simulink model "QSMC_TEST"  (R2019a)
settings: Solver=FixedStepAuto  StartTime=0.0  StopTime=10.0  FixedStep=0.02  RelTol=1e-3
settings Model: Creator=anton  LastModifiedBy=anton

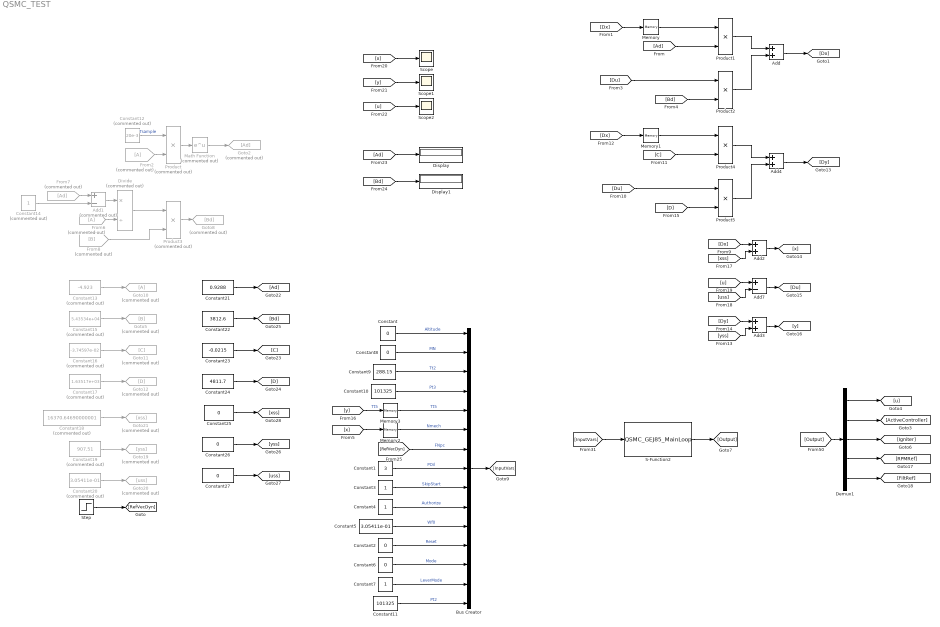
== system QSMC_TEST ==
  Add{,2..4} (4 alike) : Sum
  Add1 : Sum  Commented=on  Inputs=+-
  Add7 : Sum  Inputs=+-
  Bus Creator : BusCreator  Inputs=15
  Constant{,2,6,8,25..27} (7 alike) : Constant  Value=0
  Constant1 : Constant  Value=3
  Constant10 : Constant  Value=101325
  Constant11 : Constant  Value=101325
  Constant12 : Constant  Commented=on  Value=20e-3
  Constant13 : Constant  Commented=on  Value=-4.923
  Constant14 : Constant  Commented=on
  Constant15 : Constant  Commented=on  Value=5.43534e+04
  Constant16 : Constant  Commented=on  Value=-3.74597e-02
  Constant17 : Constant  Commented=on  Value=1.63517e+03
  Constant18 : Constant  Commented=on  Value=16370.64690000001
  Constant19 : Constant  Commented=on  Value=907.51
  Constant20 : Constant  Commented=on  Value=3.05411e-01
  Constant21 : Constant  Value=0.9288
  Constant22 : Constant  Value=3812.6
  Constant23 : Constant  Value=-0.0215
  Constant24 : Constant  Value=4811.7
  Constant3 : Constant
  Constant4 : Constant
  Constant5 : Constant  Value=3.05411e-01
  Constant7 : Constant
  Constant9 : Constant  Value=288.15
  Demux1 : Demux  Outputs=5
  Display : Display
  Display1 : Display
  Divide : Product  Commented=on  Inputs=*/
  From2 : From  Commented=on
  From6 : From  Commented=on
  From7 : From  Commented=on  GotoTag=Ad
  From8 : From  Commented=on  GotoTag=B
  Goto10 : Goto  Commented=on
  Goto11 : Goto  Commented=on  GotoTag=C
  Goto12 : Goto  Commented=on  GotoTag=D
  Goto19 : Goto  Commented=on  GotoTag=yss
  Goto2 : Goto  Commented=on  GotoTag=Ad
  Goto20 : Goto  Commented=on  GotoTag=uss
  Goto21 : Goto  Commented=on  GotoTag=xss
  Goto5 : Goto  Commented=on  GotoTag=B
  Goto8 : Goto  Commented=on  GotoTag=Bd
  Math Function : Math  Commented=on  SaturateOnIntegerOverflow=on
  Memory : Memory
  Memory1 : Memory
  Memory2 : Memory  InitialCondition=16370.64690000001
  Memory3 : Memory  InitialCondition=907.51
  Product : Product  Commented=on
  Product{1..2,4..5} (4 alike) : Product
  Product3 : Product  Commented=on
  S-Function2 : S-Function  FunctionName=QSMC_GEJ85_MainLoop  SFunctionDeploymentMode=off  EnableBusSupport=off
  Scope : Scope
  Scope1 : Scope
  Scope2 : Scope
  Step : Step  Before=1  After=0.95  SampleTime=0
  wires:
  S-Function2/1 -> [Output]
  Constant7/1 -> Bus Creator/14  "LeverMode"
  Constant2/1 -> Bus Creator/12  "Reset"
  Constant6/1 -> Bus Creator/13  "Mode"
  [y] -> Memory3/1  "Tt5"
  Demux1/2 -> [ActiveController]
  Constant10/1 -> Bus Creator/4  "Pt3"
  Constant3/1 -> Bus Creator/9  "SkipStart"
  Bus Creator/1 -> [InputVars]
  [Output] -> Demux1/1
  Constant9/1 -> Bus Creator/3  "Tt2"
  Constant4/1 -> Bus Creator/10  "Authorize"
  Demux1/1 -> [u]
  Constant8/1 -> Bus Creator/2  "MN"
  Constant1/1 -> Bus Creator/8  "POil"
  Memory2/1 -> Bus Creator/6  "Nmech"
  Constant5/1 -> Bus Creator/11  "Wf0"
  Demux1/3 -> [Igniter]
  [RefVecDyn] -> Bus Creator/7  "FNpc"
  [InputVars] -> S-Function2/1
  Demux1/4 -> [RPMRef]
  Demux1/5 -> [FiltRef]
  Constant/1 -> Bus Creator/1  "Altitude"
  Product1/1 -> Add/1
  Product2/1 -> Add/2
  Add/1 -> [Dx]
  [Dx] -> Memory/1
  [x] -> Memory2/1
  Product/1 -> Math Function/1
  Constant12/1 -> Product/1  "Tsample"
  From2/1 -> Product/2
  Math Function/1 -> Goto2/1
  [Ad] -> Product1/2
  Add1/1 -> Divide/1
  Divide/1 -> Product3/1
  From6/1 -> Divide/2
  From7/1 -> Add1/1
  Constant14/1 -> Add1/2
  From8/1 -> Product3/2
  Product3/1 -> Goto8/1
  Constant15/1 -> Goto5/1
  Constant13/1 -> Goto10/1
  [Bd] -> Product2/2
  Memory/1 -> Product1/1
  [Du] -> Product2/1
  Constant16/1 -> Goto11/1
  Constant17/1 -> Goto12/1
  [Du] -> Product5/1
  Memory1/1 -> Product4/1
  [D] -> Product5/2
  [C] -> Product4/2
  Add4/1 -> [Dy]
  Product5/1 -> Add4/2
  Product4/1 -> Add4/1
  [Dx] -> Add2/1
  [xss] -> Add2/2
  Add2/1 -> [x]
  Add7/1 -> [Du]
  [uss] -> Add7/2
  [u] -> Add7/1
  [Dx] -> Memory1/1
  Add3/1 -> [y]
  [yss] -> Add3/2
  [Dy] -> Add3/1
  Constant20/1 -> Goto20/1
  Constant19/1 -> Goto19/1
  Constant18/1 -> Goto21/1
  [x] -> Scope/1
  [y] -> Scope1/1
  [u] -> Scope2/1
  [Ad] -> Display/1
  [Bd] -> Display1/1
  Step/1 -> [RefVecDyn]
  Memory3/1 -> Bus Creator/5  "Tt5"
  Constant11/1 -> Bus Creator/15  "Pt2"
  Constant24/1 -> [D]
  Constant23/1 -> [C]
  Constant21/1 -> [Ad]
  Constant22/1 -> [Bd]
  Constant25/1 -> [xss]
  Constant26/1 -> [yss]
  Constant27/1 -> [uss]
